simulink model "GPSModel"  (R2023b)
settings: Solver=VariableStepAuto  StartTime=0.0  StopTime=106.1  RelTol=1e-3
libraries: sensorgpslib x1
settings Model: Creator=The MathWorks, Inc.  LastModifiedBy=YOUSRA
settings DebuggingCC: UnconnectedInputMsg=warning  UnconnectedOutputMsg=warning  UnconnectedLineMsg=warning
settings ModelReferenceCC: EnableRefExpFcnMdlSchedulingChecks=on
settings RTWCC: DLArmComputeVersion=19.05

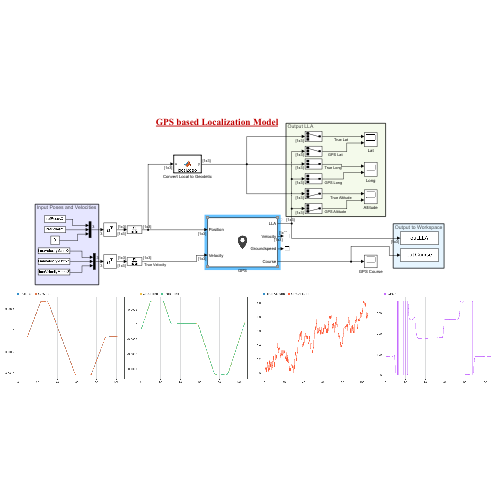
[thumbnail: Simulink's stored preview of the top-level diagram]
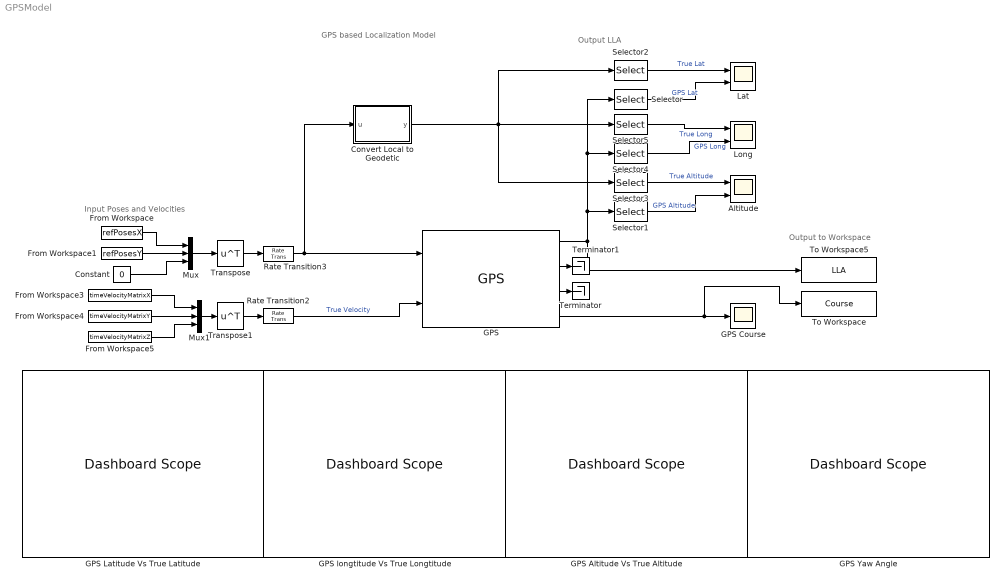
== system GPSModel ==
  note: Output to Workspace
  note: Output LLA
  note: Input Poses and Velocities
  note: GPS based Localization Model
  Altitude : Scope  NumInputPorts=2
  Constant : Constant  Value=0
  Convert Local to Geodetic : MATLAB Function  TreatAsAtomicUnit=on
  From Workspace : FromWorkspace  VariableName=refPosesX
  From Workspace1 : FromWorkspace  VariableName=refPosesY
  From Workspace3 : FromWorkspace  VariableName=timeVelocityMatrixX
  From Workspace4 : FromWorkspace  VariableName=timeVelocityMatrixY
  From Workspace5 : FromWorkspace  VariableName=timeVelocityMatrixZ
  GPS : sensorgpslib/GPS  DispRefFrame=NED  PositionInputFormat=Local  ReferenceLocation=[ 0, 0, 0]  HorizontalPositionAccuracy=0.9  VerticalPositionAccuracy=0.9  VelocityAccuracy=1  DecayFactor=0.999  SeedDouble=67  SimulateUsing=Interpreted execution
  GPS Altitude Vs True Altitude : DashboardScope
  GPS Course : Scope
  GPS Latitude Vs True Latitude : DashboardScope  Ymin=-50  Ymax=50  UpdateMode=Scroll
  GPS Yaw Angle : DashboardScope  Ymin=0  Ymax=360
  GPS longtitude Vs True Longtitude : DashboardScope
  Lat : Scope  NumInputPorts=2
  Long : Scope  NumInputPorts=2
  Mux : Mux  Inputs=3
  Mux1 : Mux  Inputs=3
  Rate Transition2 : RateTransition  OutPortSampleTime=1/4.707
  Rate Transition3 : RateTransition  OutPortSampleTime=1/4.707
  Selector : Selector  InputPortWidth=3  IndexOptions=Index vector (dialog)  Indices=[1]  OutputSizes=1
  Selector1 : Selector  InputPortWidth=3  IndexOptions=Index vector (dialog)  Indices=[3]  OutputSizes=1
  Selector2 : Selector  InputPortWidth=3  IndexOptions=Index vector (dialog)  Indices=[1]  OutputSizes=1
  Selector3 : Selector  InputPortWidth=3  IndexOptions=Index vector (dialog)  Indices=[3]  OutputSizes=1
  Selector4 : Selector  InputPortWidth=3  IndexOptions=Index vector (dialog)  Indices=[2]  OutputSizes=1
  Selector5 : Selector  InputPortWidth=3  IndexOptions=Index vector (dialog)  Indices=[2]  OutputSizes=1
  Terminator : Terminator
  Terminator1 : Terminator
  To Workspace : ToWorkspace  VariableName=Course  SaveFormat=Timeseries  SampleTime=-1
  To Workspace5 : ToWorkspace  VariableName=LLA  SaveFormat=Timeseries  SampleTime=-1
  Transpose : Math  Operator=transpose
  Transpose1 : Math  Operator=transpose
  wires:
  GPS/4 -> To Workspace/1, GPS Course/1
  GPS/1 -> Selector1/1, Selector/1, Selector4/1, To Workspace5/1
  From Workspace/1 -> Mux/1
  Mux/1 -> Transpose/1
  From Workspace3/1 -> Mux1/1
  Mux1/1 -> Transpose1/1
  Transpose1/1 -> Rate Transition2/1
  Rate Transition2/1 -> GPS/2  "True Velocity"
  Transpose/1 -> Rate Transition3/1
  Selector/1 -> Lat/2  "GPS Lat"
  Selector2/1 -> Lat/1  "True Lat"
  Selector3/1 -> Altitude/1  "True Altitude"
  Selector1/1 -> Altitude/2  "GPS Altitude"
  From Workspace1/1 -> Mux/2
  Constant/1 -> Mux/3
  From Workspace4/1 -> Mux1/2
  From Workspace5/1 -> Mux1/3
  Selector5/1 -> Long/1  "True Long"
  Selector4/1 -> Long/2  "GPS Long"
  GPS/3 -> Terminator/1
  GPS/2 -> Terminator1/1
  Rate Transition3/1 -> GPS/1, Convert Local to Geodetic/1(u)
  Convert Local to Geodetic/1(y) -> Selector3/1, Selector5/1, Selector2/1

== matlab function GPSModel/Convert Local to Geodetic ==
  data: u input; y output
function y = local2geo(u)

y = ned2lla(u,[0 0 0],"ellipsoid");

end
